simulink model "FrictionModel_Switch_Final_ROA"  (R2018b)
settings: Solver=VariableStepAuto  StartTime=0.0  StopTime=20  RelTol=1e-3
values from neighbouring files (symbols this model uses):
  C1 = (2/Cprime)^2    (= 0.00510204081633)    [Friction_Switch_FinalReport.m]
  C2 = 4/Cprime    (= 0.142857142857)    [Friction_Switch_FinalReport.m]
  ce = (min(eig(P)))*cc    [Friction_Switch_FinalReport.m]
  k = place(Amat,Bmat,spoles)    [Friction_Switch_FinalReport.m]
  KM = ((Cprime/2)^2)/D    (= 0.0834042553191)    [Friction_Switch_FinalReport.m]
  P = lyap((a_2-b_2*k_2)',eye(2))    [Friction_Switch_FinalReport.m]
settings Model: Creator=rob  LastModifiedBy=BSR
settings SFSimCC: SimUseLocalCustomCode=off
settings RTWCC: RTWUseLocalCustomCode=off

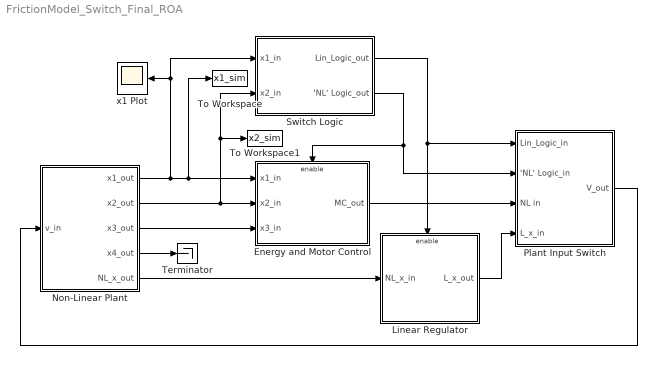
== system FrictionModel_Switch_Final_ROA ==
  Energy and Motor Control : Subsystem
  Linear Regulator : Subsystem
  Non-Linear Plant : Subsystem
  Plant Input Switch : Subsystem
  Switch Logic : Subsystem
  Terminator : Terminator
  To Workspace : ToWorkspace  VariableName=x1_sim  SampleTime=-1
      settings: Save2DSignal=2-D array (concatenate along first dimension)
  To Workspace1 : ToWorkspace  VariableName=x2_sim  SampleTime=-1
      settings: Save2DSignal=2-D array (concatenate along first dimension)
  x1 Plot : Scope
  wires:
  Switch Logic/1(Lin_Logic_out) -> Linear Regulator/Enable, Plant Input Switch/1(Lin_Logic_in)
  Switch Logic/2('NL' Logic_out) -> Energy and Motor Control/Enable, Plant Input Switch/2('NL' Logic_in)
  Energy and Motor Control/1(MC_out) -> Plant Input Switch/3(NL in)
  Linear Regulator/1(L_x_out) -> Plant Input Switch/4(L_x_in)
  Plant Input Switch/1(V_out) -> Non-Linear Plant/1(v_in)
  Non-Linear Plant/5(NL_x_out) -> Linear Regulator/1(NL_x_in)
  Non-Linear Plant/1(x1_out) -> x1 Plot/1, Switch Logic/1(x1_in), To Workspace/1, Energy and Motor Control/1(x1_in)
  Non-Linear Plant/2(x2_out) -> Switch Logic/2(x2_in), To Workspace1/1, Energy and Motor Control/2(x2_in)
  Non-Linear Plant/3(x3_out) -> Energy and Motor Control/3(x3_in)
  Non-Linear Plant/4(x4_out) -> Terminator/1

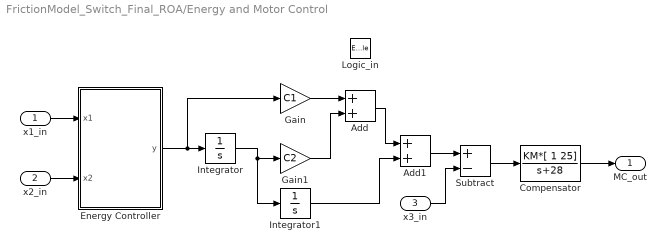
== system FrictionModel_Switch_Final_ROA/Energy and Motor Control ==
  x1_in : Inport
  x2_in : Inport  Port=2
  x3_in : Inport  Port=3
  Logic_in : EnablePort
  Add : Sum
  Add1 : Sum
  Compensator : TransferFcn  Numerator=KM*[ 1 25]  Denominator=[1 28]
  Energy Controller : MATLAB Function  TreatAsAtomicUnit=on
  Gain : Gain  Gain=C1
  Gain1 : Gain  Gain=C2
  Integrator : Integrator
  Integrator1 : Integrator
  Subtract : Sum  Inputs=+-
  MC_out : Outport
  wires:
  Gain1/1 -> Add/2
  Add/1 -> Add1/1
  Integrator1/1 -> Add1/2
  Add1/1 -> Subtract/1
  Subtract/1 -> Compensator/1
  Energy Controller/1(y) -> Integrator/1, Gain/1
  Integrator/1 -> Integrator1/1, Gain1/1
  Gain/1 -> Add/1
  Compensator/1 -> MC_out/1
  x1_in/1 -> Energy Controller/1(x1)
  x3_in/1 -> Subtract/2
  x2_in/1 -> Energy Controller/2(x2)

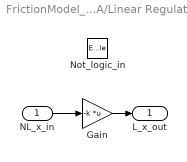
== system FrictionModel_Switch_Final_ROA/Linear Regulator ==
  NL_x_in : Inport
  Not_logic_in : EnablePort
  Gain : Gain  Gain=-k  Multiplication=Matrix(K*u)
  L_x_out : Outport
  wires:
  NL_x_in/1 -> Gain/1
  Gain/1 -> L_x_out/1

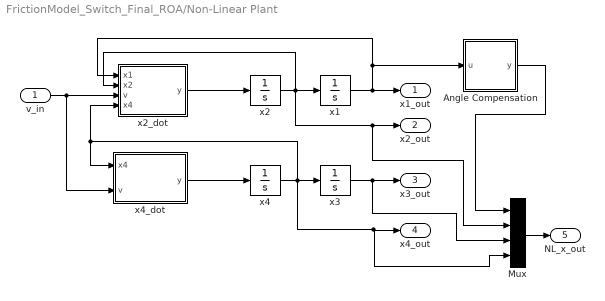
== system FrictionModel_Switch_Final_ROA/Non-Linear Plant ==
  v_in : Inport
  Angle Compensation : MATLAB Function  TreatAsAtomicUnit=on
  Mux : Mux
  x1 : Integrator  InitialCondition=pi
  x2 : Integrator  InitialCondition=0.2
  x2_dot : MATLAB Function  TreatAsAtomicUnit=on
  x3 : Integrator
  x4 : Integrator
  x4_dot : MATLAB Function  TreatAsAtomicUnit=on
  x1_out : Outport
  x2_out : Outport  Port=2
  x3_out : Outport  Port=3
  x4_out : Outport  Port=4
  NL_x_out : Outport  Port=5
  wires:
  v_in/1 -> x4_dot/2(v), x2_dot/3(v)
  x2/1 -> x2_dot/2(x2), Mux/2, x2_out/1, x1/1
  x4_dot/1(y) -> x4/1
  x4/1 -> x3/1, x4_out/1, Mux/4, x2_dot/4(x4), x4_dot/1(x4)
  x3/1 -> Mux/3, x3_out/1
  Mux/1 -> NL_x_out/1
  x2_dot/1(y) -> x2/1
  x1/1 -> x2_dot/1(x1), Angle Compensation/1(u), x1_out/1
  Angle Compensation/1(y) -> Mux/1

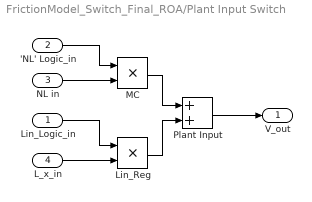
== system FrictionModel_Switch_Final_ROA/Plant Input Switch ==
  Lin_Logic_in : Inport
  'NL' Logic_in : Inport  Port=2
  NL in : Inport  Port=3
  L_x_in : Inport  Port=4
  Lin_Reg : Product
  MC : Product
  Plant Input : Sum
  V_out : Outport
  wires:
  'NL' Logic_in/1 -> MC/1
  MC/1 -> Plant Input/1
  L_x_in/1 -> Lin_Reg/2
  NL in/1 -> MC/2
  Lin_Reg/1 -> Plant Input/2
  Plant Input/1 -> V_out/1
  Lin_Logic_in/1 -> Lin_Reg/1

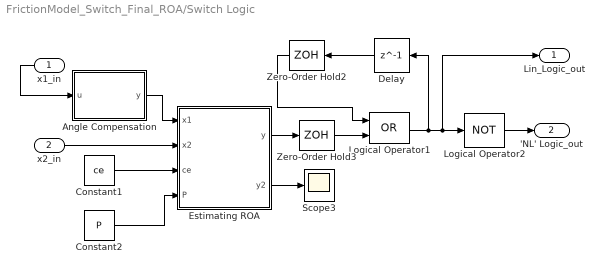
== system FrictionModel_Switch_Final_ROA/Switch Logic ==
  x1_in : Inport
  x2_in : Inport  Port=2
  Angle Compensation : MATLAB Function  TreatAsAtomicUnit=on
  Constant1 : Constant  Value=ce
  Constant2 : Constant  Value=P
  Delay : Delay  DelayLength=1
  Estimating ROA : MATLAB Function  TreatAsAtomicUnit=on
  Logical Operator1 : Logic  Operator=OR  AllPortsSameDT=off  OutDataTypeStr=boolean
  Logical Operator2 : Logic  Operator=NOT  AllPortsSameDT=off  OutDataTypeStr=boolean
  Scope3 : Scope
  Zero-Order Hold2 : ZeroOrderHold  SampleTime=0.001
  Zero-Order Hold3 : ZeroOrderHold  SampleTime=0.001
  Lin_Logic_out : Outport
  'NL' Logic_out : Outport  Port=2
  wires:
  x1_in/1 -> Angle Compensation/1(u)
  x2_in/1 -> Estimating ROA/2(x2)
  Constant1/1 -> Estimating ROA/3(ce)
  Constant2/1 -> Estimating ROA/4(P)
  Logical Operator1/1 -> Logical Operator2/1, Lin_Logic_out/1, Delay/1
  Logical Operator2/1 -> 'NL' Logic_out/1
  Estimating ROA/2(y2) -> Scope3/1
  Estimating ROA/1(y) -> Zero-Order Hold3/1
  Zero-Order Hold3/1 -> Logical Operator1/2
  Delay/1 -> Zero-Order Hold2/1
  Zero-Order Hold2/1 -> Logical Operator1/1
  Angle Compensation/1(y) -> Estimating ROA/1(x1)

== matlab function FrictionModel_Switch_Final_ROA/Switch Logic/Estimating ROA ==
  data: x1 input; y output; x2 input; ce input; P input; y2 output
function [y,y2] = fcn(x1,x2,ce,P)
y2 = [x1; x2]'*P*[x1; x2];
if y2 < ce
   y=1;
else
    y = 0;
end

== matlab function FrictionModel_Switch_Final_ROA/Non-Linear Plant/x2_dot ==
  data: x1 input; x2 input; v input; y output; x4 input
function y = fcn(x1, x2, v, x4)
A=22.8;
g=9.8;
D=2350;
n=495;
c=25;
alpha=0.018;
u= (A*sin(x1))-(((A/g)*cos(x1))*((-c*x4)+(D*v))/n)-(alpha*(x2^2)*sign(x2));
y = u;

== matlab function FrictionModel_Switch_Final_ROA/Non-Linear Plant/x4_dot ==
  data: x4 input; v input; y output
function y = fcn(x4, v)
D=2350;
c=25;
u= (D*v)-(c*x4);
y = u;

== matlab function FrictionModel_Switch_Final_ROA/Energy and Motor Control/Energy Controller ==
  data: x1 input; y output; x2 input
function y  = fcn(x1, x2)
A = 22.8;%Square of natural frequency of pendulum
g=9.81;%Gravity
n=495;% Transduction ratio to the lead screw
k = 0.02; %Gain for Energy System (User input) orignal = 0.016
alpha=0.018; %Co-efficient of friction (User input)original=0.04
E = 0.5*(x2^2)+A*(cos(x1)-1); %Enery of the pendulum system
if abs(cos(x1)) < 0.08 % This will account for when cos(X1)is close to 0
    w = 0.08*sign(cos(x1));
else 
    w=cos(x1);
end
u1 = (1)*(k*E*x2*cos(x1))-((g/A)*alpha*(x2^2)*(sign(x2))/w); %Pivot acc.
u=u1*n; % We need to convert account for our transducer ratio
vdot = E*((alpha*(x2^2)*sign(x2))-((A/g)*x2*cos(x1)*u1));
y = u;

== matlab function FrictionModel_Switch_Final_ROA/Non-Linear Plant/Angle Compensation ==
  data: u input; y output
function y = fcn(u)
if u > pi
    y = (u - 2*pi);  
else
y = u;
end

== matlab function FrictionModel_Switch_Final_ROA/Switch Logic/Angle Compensation ==
  data: u input; y output
function y = fcn(u)

if u > pi
    y = abs(u - 2*pi);
    
else
  
y = u;
end
